simulink model "gm_sampleModel1489_1_sub_sub"  (R2023a)
settings: Solver=VariableStepAuto  StartTime=0.0  StopTime=10.0  RelTol=1e-3
libraries: hdlsllib x5, simulink x1
settings Model: Creator=user1  LastModifiedBy=user1
settings OptimizationCC: BlockReduction=off  ConditionallyExecuteInputs=off
settings DebuggingCC: InheritedTsInSrcMsg=none

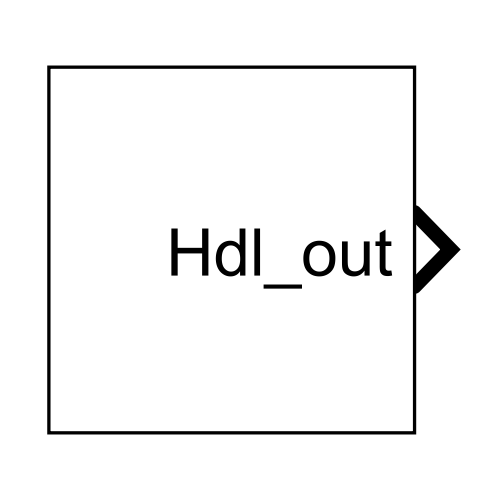
[thumbnail: Simulink's stored preview of the top-level diagram]
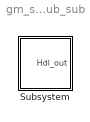
== system gm_sampleModel1489_1_sub_sub ==
  Subsystem : Subsystem

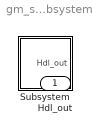
== system gm_sampleModel1489_1_sub_sub/Subsystem ==
  Subsystem : Subsystem
  Hdl_out : Outport  OutDataTypeStr=uint8

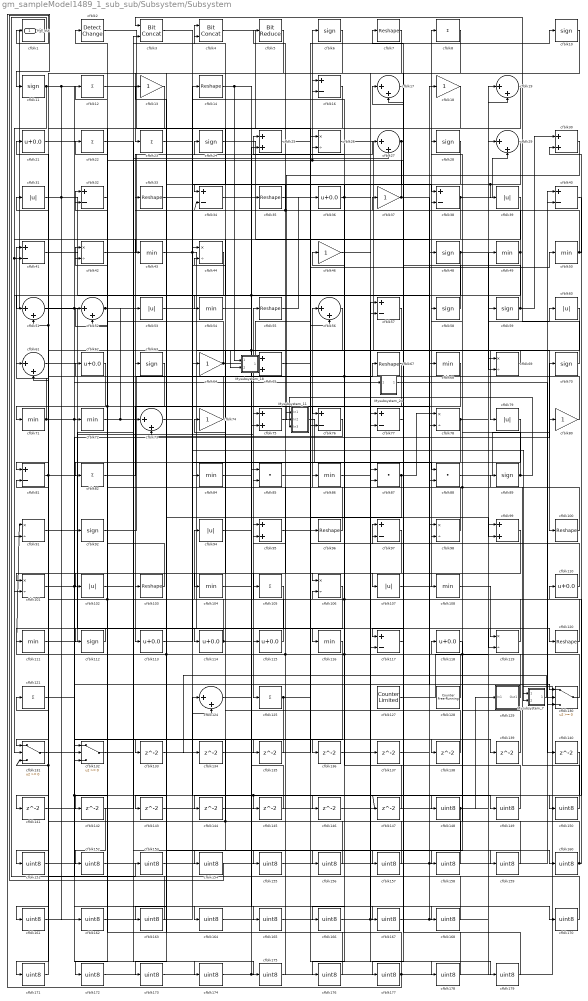
== system gm_sampleModel1489_1_sub_sub/Subsystem/Subsystem ==
  Mysubsystem_11 : Subsystem  TreatAsAtomicUnit=on  RTWFcnName=Mysubsystem_11
      settings: RTWFcnNameOpts=User specified  RTWFileNameOpts=Use function name
  Mysubsystem_18 : Subsystem  TreatAsAtomicUnit=on  RTWFcnName=Mysubsystem_18
      settings: RTWFcnNameOpts=User specified  RTWFileNameOpts=Use function name
  Mysubsystem_24 : Subsystem  TreatAsAtomicUnit=on  RTWFcnName=Mysubsystem_24
      settings: RTWFcnNameOpts=User specified  RTWFileNameOpts=Use function name
  Mysubsystem_7 : Subsystem  TreatAsAtomicUnit=on  RTWFcnName=Mysubsystem_7
      settings: RTWFcnNameOpts=User specified  RTWFileNameOpts=Use function name
  cfblk1 : ArithShift  BitShiftNumber=8
  cfblk{6,10..11,24,28,48,58..59,63,70,89,92,112} (13 alike) : Signum
  cfblk{7,14,33,35,55,67,96,100,103,120} (10 alike) : Reshape
  cfblk{26,42,44,69,78,91,98,101,106,119} (10 alike) : Product  Inputs=*/  OutDataTypeStr=uint8  RndMeth=Zero  SaturateOnIntegerOverflow=on
  cfblk{31,39,53,60,79,94,102,107} (8 alike) : Abs  OutDataTypeStr=uint8  SaturateOnIntegerOverflow=off
  cfblk{43,49..50,54,68,71..72,84,86,104,108,111,116} (13 alike) : MinMax  OutDataTypeStr=uint8
  cfblk{8,12,22..23,82,105,121,125} (8 alike) : Sum  Inputs=+  OutDataTypeStr=uint8
  cfblk{21,36,62,110,113..115,118} (8 alike) : Bias  Bias=0.0  SaturateOnIntegerOverflow=off
  cfblk{16,32,34,38,40..41,57,76..77,81,97,117} (12 alike) : Sum  Inputs=+-  OutDataTypeStr=uint8
  cfblk{17,19,27,29,51..52,56,61,73,124} (10 alike) : Sum  Inputs=|++  OutDataTypeStr=uint8
  cfblk127 : hdlsllib/Sources/Counter Limited  uplimit=7  tsamp=-1
  cfblk128 : hdlsllib/Sources/Counter Free-Running  NumBits=16  tsamp=-1
  cfblk129 : Subsystem
      settings: LibrarySourceBlock=|
      | hdlsllib/Ports &
      | Subsystems/Subsystem
  cfblk{13,18,37,46,64,74,80} (7 alike) : Gain  OutDataTypeStr=uint8
  cfblk130 : Switch  OutDataTypeStr=uint8  SaturateOnIntegerOverflow=off  InputSameDT=off
  cfblk131 : Switch  OutDataTypeStr=uint8  SaturateOnIntegerOverflow=off  InputSameDT=off
  cfblk132 : Switch  OutDataTypeStr=uint8  SaturateOnIntegerOverflow=off  InputSameDT=off
  cfblk{133..147} (15 alike) : Delay  SampleTime=1
  cfblk{148..168,170..179} (31 alike) : DataTypeConversion  OutDataTypeStr=uint8  SaturateOnIntegerOverflow=off  RndMeth=Floor
  cfblk2 : simulink/Logic and Bit Operations/Detect Change  vinit=0  OutDataTypeStr=uint8
      settings: LibrarySourceBlock=|
      | hdlsllib/Logic and Bit
      | Operations/Detect
      | Change
  cfblk{25,30,65,75,95,99} (6 alike) : Sum  OutDataTypeStr=uint8
  cfblk3 : hdlsllib/Logic and Bit Operations/Bit Concat  numInputs=2
  cfblk4 : hdlsllib/Logic and Bit Operations/Bit Concat  numInputs=2
  cfblk5 : hdlsllib/Logic and Bit Operations/Bit Reduce  mode=AND
  cfblk85 : DotProduct  OutDataTypeStr=uint8
  cfblk87 : DotProduct  OutDataTypeStr=uint8
  cfblk88 : DotProduct  OutDataTypeStr=uint8
  Hdl_out : Outport  OutDataTypeStr=uint8
  wires:
  cfblk53/1 -> cfblk116/1
  cfblk110/1 -> cfblk97/1
  cfblk115/1 -> cfblk55/1
  cfblk128/1 -> cfblk95/2, cfblk91/1
  cfblk55/1 -> cfblk36/1
  cfblk80/1 -> cfblk42/1, cfblk25/1
  cfblk92/1 -> cfblk67/1
  cfblk82/1 -> cfblk24/1
  cfblk26/1 -> cfblk79/1
  cfblk107/1 -> cfblk8/1
  cfblk127/1 -> cfblk59/1
  cfblk5/1 -> cfblk23/1
  cfblk67/1 -> cfblk113/1
  cfblk27/1 -> cfblk105/1, cfblk117/1
  cfblk39/1 -> cfblk41/2, cfblk91/2
  cfblk96/1 -> cfblk56/1
  cfblk103/1 -> cfblk2/1
  cfblk51/1 -> cfblk114/1, Mysubsystem_24/1(In1)
  cfblk4/1 -> cfblk96/1
  cfblk23/1 -> cfblk88/1
  cfblk36/1 -> cfblk178/1, cfblk106/1
  cfblk2/1 -> cfblk64/1
  cfblk16/1 -> cfblk34/1
  cfblk12/1 -> cfblk56/2
  cfblk43/1 -> cfblk16/1, cfblk100/1
  cfblk71/1 -> cfblk165/1, cfblk41/1
  cfblk70/1 -> cfblk3/1
  cfblk120/1 -> cfblk46/1, cfblk61/1
  cfblk54/1 -> cfblk120/1
  cfblk108/1 -> cfblk119/1
  cfblk50/1 -> cfblk30/2, cfblk34/2, cfblk5/1
  cfblk100/1 -> cfblk4/2, cfblk28/1
  cfblk130/1 -> cfblk32/2, cfblk63/1
  cfblk64/1 -> cfblk42/2, cfblk50/1
  cfblk24/1 -> cfblk108/1
  cfblk65/1 -> cfblk10/1
  cfblk88/1 -> cfblk70/1
  cfblk42/1 -> cfblk27/1
  cfblk125/1 -> cfblk179/1, cfblk144/1
  cfblk31/1 -> cfblk162/1, cfblk98/1
  cfblk44/1 -> cfblk71/1
  cfblk87/1 -> cfblk78/1, cfblk103/1
  cfblk99/1 -> cfblk125/1
  cfblk113/1 -> cfblk14/1
  cfblk63/1 -> cfblk142/1, cfblk141/1
  cfblk33/1 -> cfblk38/1
  cfblk68/1 -> cfblk166/1
  cfblk21/1 -> cfblk136/1, cfblk72/1
  cfblk72/1 -> cfblk53/1, cfblk76/1
  cfblk101/1 -> cfblk130/2, cfblk75/1
  cfblk102/1 -> cfblk73/1
  cfblk77/1 -> cfblk7/1
  cfblk14/1 -> cfblk69/2, cfblk78/2, Mysubsystem_18/1(In1)
  cfblk59/1 -> cfblk30/1, cfblk33/1
  cfblk129/1(Out1) -> cfblk58/1, cfblk16/2, cfblk95/1
  cfblk6/1 -> cfblk81/1
  cfblk94/1 -> cfblk25/2
  cfblk75/1 -> cfblk117/2
  cfblk114/1 -> cfblk139/1, cfblk32/1, cfblk61/2
  cfblk111/1 -> cfblk4/1
  cfblk112/1 -> cfblk111/1
  cfblk46/1 -> cfblk119/2
  cfblk52/1 -> Hdl_out/1, cfblk155/1
  cfblk95/1 -> cfblk97/2
  cfblk124/1 -> cfblk160/1
  cfblk17/1 -> cfblk177/1
  cfblk25/1 -> cfblk76/2
  cfblk81/1 -> cfblk101/1, cfblk27/2
  cfblk119/1 -> cfblk94/1
  cfblk49/1 -> cfblk37/1, cfblk132/3
  cfblk32/1 -> cfblk82/1
  cfblk48/1 -> cfblk69/1, cfblk65/2, cfblk131/2
  cfblk13/1 -> cfblk112/1
  cfblk35/1 -> cfblk99/2
  cfblk76/1 -> cfblk73/2
  cfblk131/1 -> cfblk80/1
  cfblk38/1 -> cfblk54/1, cfblk29/2
  cfblk86/1 -> cfblk148/1
  cfblk74/1 -> cfblk51/2, cfblk31/1
  cfblk41/1 -> cfblk84/1
  cfblk98/1 -> cfblk62/1
  cfblk19/1 -> cfblk172/1
  cfblk60/1 -> cfblk104/1
  cfblk91/1 -> cfblk115/1
  cfblk37/1 -> cfblk130/1, cfblk12/1, cfblk6/1
  cfblk89/1 -> cfblk38/2, Mysubsystem_11/3(In3)
  cfblk8/1 -> cfblk77/2
  cfblk56/1 -> cfblk131/1
  cfblk78/1 -> cfblk60/1, cfblk102/1
  cfblk11/1 -> cfblk101/2, cfblk92/1, cfblk174/1, cfblk147/1, cfblk145/1
  cfblk7/1 -> cfblk43/1
  cfblk29/1 -> cfblk133/1, cfblk39/1
  cfblk10/1 -> cfblk107/1
  cfblk34/1 -> cfblk35/1
  cfblk58/1 -> cfblk26/2
  cfblk18/1 -> cfblk51/1
  cfblk133/1 -> cfblk26/1
  cfblk116/1 -> cfblk135/1
  cfblk135/1 -> cfblk132/2
  cfblk136/1 -> cfblk87/2
  cfblk137/1 -> cfblk88/2
  cfblk61/1 -> cfblk138/1
  cfblk138/1 -> cfblk44/1
  cfblk139/1 -> cfblk98/2
  cfblk141/1 -> cfblk3/2
  cfblk105/1 -> cfblk143/1
  cfblk143/1 -> cfblk29/1
  cfblk144/1 -> cfblk99/1
  cfblk145/1 -> cfblk65/1
  cfblk104/1 -> cfblk146/1
  cfblk146/1 -> cfblk77/1
  cfblk147/1 -> cfblk106/2
  cfblk148/1 -> cfblk173/1, cfblk129/1(In1)
  cfblk3/1 -> cfblk149/1
  cfblk149/1 -> cfblk86/1
  cfblk40/1 -> cfblk150/1
  cfblk150/1 -> cfblk89/1
  cfblk62/1 -> cfblk151/1
  cfblk151/1 -> cfblk40/1
  cfblk142/1 -> cfblk152/1
  cfblk152/1 -> cfblk40/2
  cfblk1/1 -> cfblk153/1
  cfblk153/1 -> cfblk87/1
  cfblk140/1 -> cfblk154/1
  cfblk154/1 -> cfblk1/1
  cfblk155/1 -> cfblk18/1, cfblk130/3
  cfblk28/1 -> cfblk156/1
  cfblk156/1 -> cfblk52/1
  cfblk117/1 -> cfblk157/1
  cfblk157/1 -> cfblk52/2
  cfblk118/1 -> cfblk158/1
  cfblk158/1 -> cfblk74/1
  cfblk85/1 -> cfblk159/1
  cfblk159/1 -> cfblk118/1
  cfblk160/1 -> cfblk110/1, cfblk44/2, cfblk81/2, cfblk131/3
  cfblk106/1 -> cfblk161/1
  cfblk161/1 -> cfblk124/1
  cfblk162/1 -> cfblk124/2
  cfblk57/1 -> cfblk163/1
  cfblk163/1 -> cfblk21/1
  cfblk132/1 -> cfblk164/1
  cfblk164/1 -> cfblk57/1
  cfblk165/1 -> cfblk57/2
  cfblk166/1 -> cfblk137/1, cfblk49/1, cfblk48/1
  cfblk84/1 -> cfblk167/1
  cfblk167/1 -> cfblk68/1
  cfblk134/1 -> cfblk168/1
  cfblk168/1 -> cfblk85/1
  cfblk121/1 -> cfblk170/1
  cfblk170/1 -> cfblk132/1
  cfblk97/1 -> cfblk171/1
  cfblk171/1 -> cfblk121/1
  cfblk172/1 -> cfblk75/2, Mysubsystem_7/2(In2)
  cfblk173/1 -> cfblk19/1
  cfblk174/1 -> cfblk19/2
  cfblk22/1 -> cfblk175/1
  cfblk175/1 -> cfblk85/2
  cfblk79/1 -> cfblk176/1
  cfblk176/1 -> cfblk22/1
  cfblk177/1 -> cfblk13/1, cfblk11/1
  cfblk178/1 -> cfblk17/1
  cfblk179/1 -> cfblk17/2
  cfblk73/1 -> Mysubsystem_7/1(In1)
  Mysubsystem_7/1(Out1) -> cfblk134/1
  cfblk30/1 -> Mysubsystem_11/1(In1)
  cfblk69/1 -> Mysubsystem_18/2(In2)
  Mysubsystem_18/1(Out1) -> Mysubsystem_11/2(In2)
  Mysubsystem_24/1(Out1) -> cfblk140/1

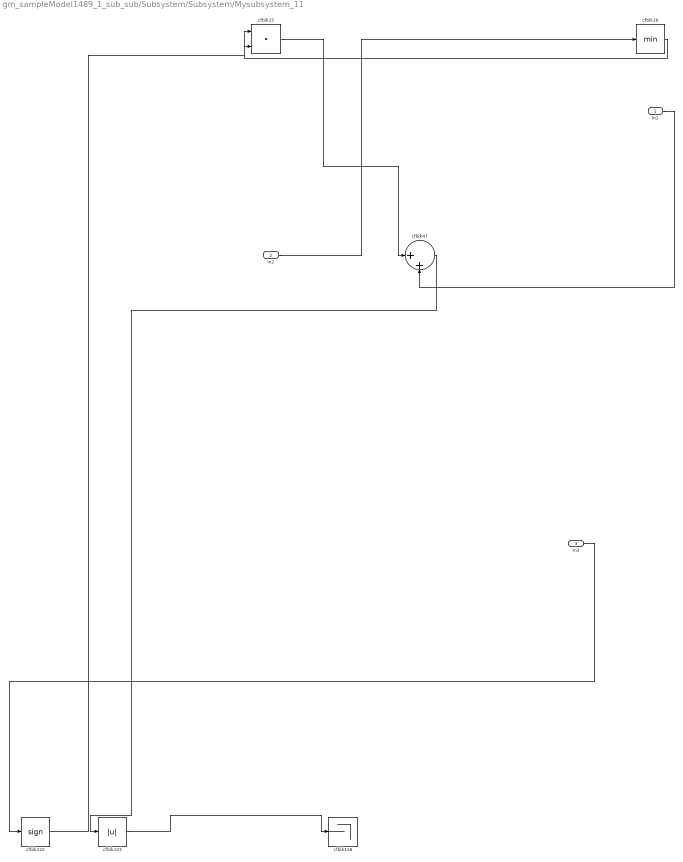
== system gm_sampleModel1489_1_sub_sub/Subsystem/Subsystem/Mysubsystem_11 ==
  In1 : Inport
  In2 : Inport  Port=2
  In3 : Inport  Port=3
  cfblk122 : Signum
  cfblk123 : Abs  SaturateOnIntegerOverflow=off
  cfblk126 : Terminator
  cfblk15 : DotProduct  OutDataTypeStr=Inherit: Inherit via internal rule
  cfblk20 : MinMax
  cfblk47 : Sum  Inputs=|++
  wires:
  In2/1 -> cfblk20/1
  cfblk122/1 -> cfblk15/1
  cfblk15/1 -> cfblk47/1
  In3/1 -> cfblk122/1
  cfblk20/1 -> cfblk15/2
  cfblk123/1 -> cfblk126/1
  In1/1 -> cfblk47/2
  cfblk47/1 -> cfblk123/1

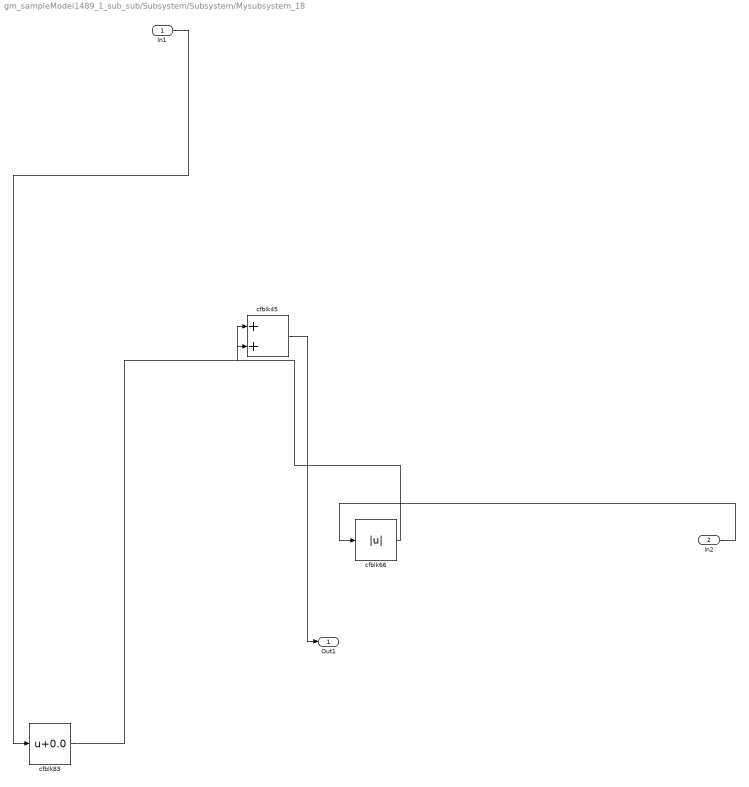
== system gm_sampleModel1489_1_sub_sub/Subsystem/Subsystem/Mysubsystem_18 ==
  In1 : Inport
  In2 : Inport  Port=2
  cfblk45 : Sum
  cfblk66 : Abs  SaturateOnIntegerOverflow=off
  cfblk83 : Bias  Bias=0.0  SaturateOnIntegerOverflow=off
  Out1 : Outport
  wires:
  cfblk45/1 -> Out1/1
  cfblk83/1 -> cfblk45/2
  In1/1 -> cfblk83/1
  cfblk66/1 -> cfblk45/1
  In2/1 -> cfblk66/1

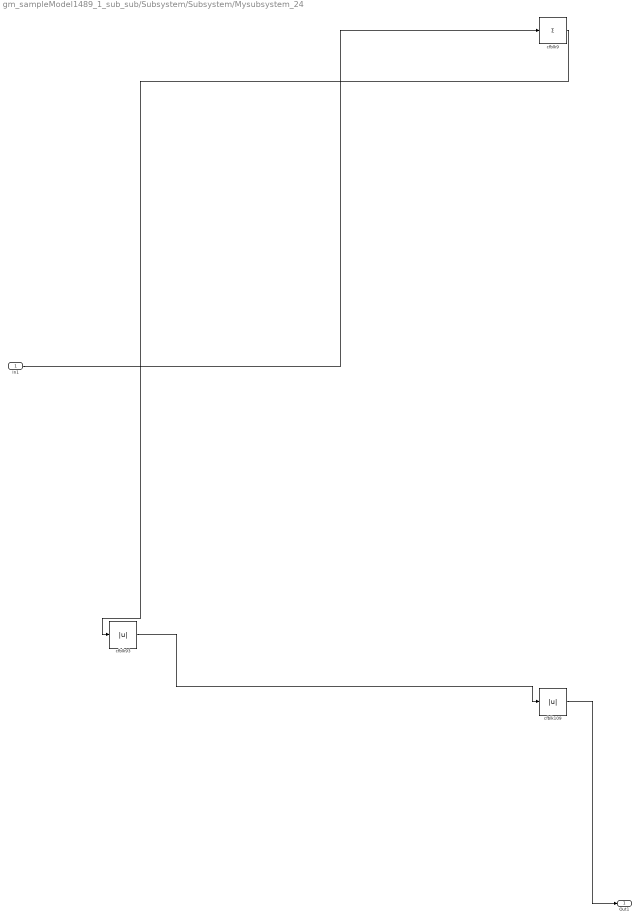
== system gm_sampleModel1489_1_sub_sub/Subsystem/Subsystem/Mysubsystem_24 ==
  In1 : Inport
  cfblk109 : Abs  SaturateOnIntegerOverflow=off
  cfblk9 : Sum  Inputs=+
  cfblk93 : Abs  SaturateOnIntegerOverflow=off
  Out1 : Outport
  wires:
  In1/1 -> cfblk9/1
  cfblk109/1 -> Out1/1
  cfblk93/1 -> cfblk109/1
  cfblk9/1 -> cfblk93/1

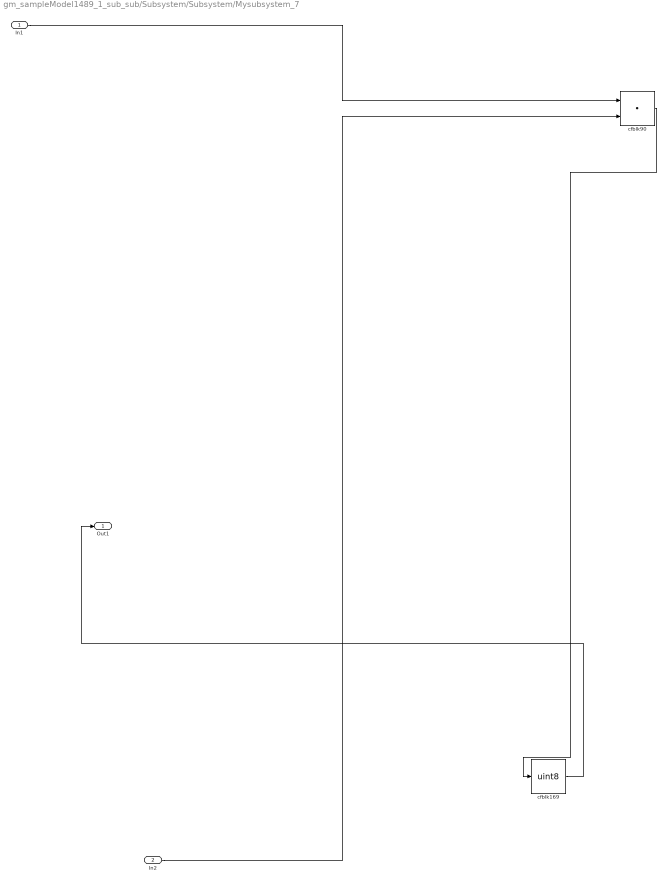
== system gm_sampleModel1489_1_sub_sub/Subsystem/Subsystem/Mysubsystem_7 ==
  In1 : Inport
  In2 : Inport  Port=2
  cfblk169 : DataTypeConversion  OutDataTypeStr=uint8  SaturateOnIntegerOverflow=off  RndMeth=Floor
  cfblk90 : DotProduct  OutDataTypeStr=Inherit: Inherit via internal rule
  Out1 : Outport
  wires:
  In1/1 -> cfblk90/1
  In2/1 -> cfblk90/2
  cfblk169/1 -> Out1/1
  cfblk90/1 -> cfblk169/1

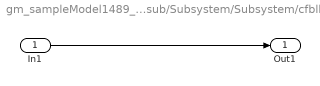
== system gm_sampleModel1489_1_sub_sub/Subsystem/Subsystem/cfblk129 ==
  In1 : Inport
  Out1 : Outport
  wires:
  In1/1 -> Out1/1
